simulink model "OPAMPs_SIMULINK"  (R2023a)
settings: Solver=VariableStepAuto  StartTime=0.0  StopTime=10.0  RelTol=1e-3
values from neighbouring files (symbols this model uses):
  C1 = 100e-9    (= 1e-07)    [ODE_OPAMPs.m]    (also in Parametros_OPAMPs.m)
  C2 = 100e-9    (= 1e-07)    [ODE_OPAMPs.m]    (also in Parametros_OPAMPs.m)
  R1 = 5e6    (= 5000000)    [ODE_OPAMPs.m]    (also in Parametros_OPAMPs.m)
  R2 = 5e6    (= 5000000)    [ODE_OPAMPs.m]    (also in Parametros_OPAMPs.m)
  R3 = 5e6    (= 5000000)    [ODE_OPAMPs.m]    (also in Parametros_OPAMPs.m)
settings Model: Creator=eveli  LastModifiedBy=eveli

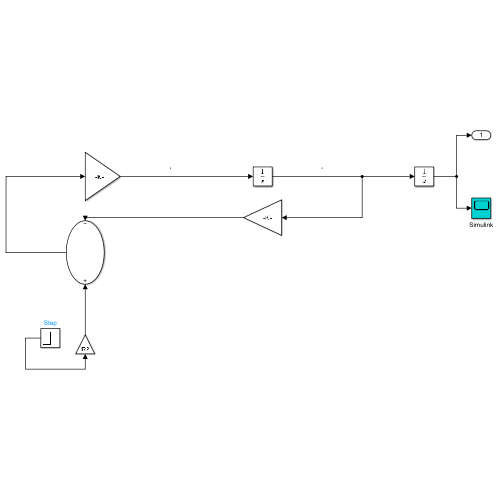
[thumbnail: Simulink's stored preview of the top-level diagram]
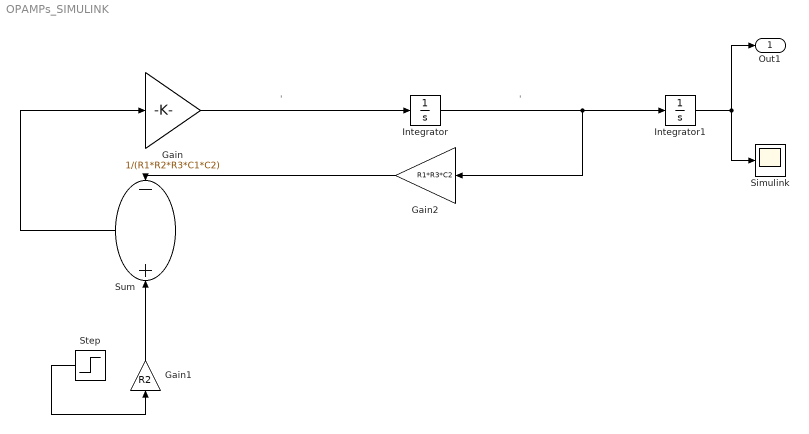
== system OPAMPs_SIMULINK ==
  note: '
  note: '
  Gain : Gain  Gain=1/(R1*R2*R3*C1*C2)
  Gain1 : Gain  Gain=R2
  Gain2 : Gain  Gain=R1*R3*C2
  Integrator : Integrator
  Integrator1 : Integrator
  Simulink : Scope
  Step : Step  Time=0  SampleTime=0
  Sum : Sum  Inputs=-+
  Out1 : Outport
  wires:
  Integrator/1 -> Gain2/1, Integrator1/1
  Gain/1 -> Integrator/1
  Step/1 -> Gain1/1
  Sum/1 -> Gain/1
  Gain2/1 -> Sum/1
  Integrator1/1 -> Simulink/1, Out1/1
  Gain1/1 -> Sum/2
